simulink model "DCM_speed_control"  (Simulink 7.6)
settings: Solver=ode23tb  StartTime=0.0  StopTime=30  FixedStep=0.0005  MaxStep=1e-4  RelTol=1e-3
values from neighbouring files (symbols this model uses):
  Bm = 0.634    [para_dc.m]
  J = 2.83    [para_dc.m]
  kphi = 4.212    [para_dc.m]
  La = .0065    (= 0.0065)    [para_dc.m]
  Ra = .066    (= 0.066)    [para_dc.m]
  TL = 0    [para_dc.m]
libraries: powerlib_extras x1
settings Model: Creator=DELL  LastModifiedBy=Rhoever  ExtModeTrigMode=oneshot  ExtModeArmWhenConnect=off
settings SolverCC: InitialStep=0.00001
settings DataIOCC: LimitDataPoints=off  SignalLoggingName=sigsOut
settings OptimizationCC: BooleanDataType=off  InitFltsAndDblsToZero=on
settings DebuggingCC: SaveWithParameterizedLinksMsg=none  SignalResolutionControl=TryResolveAllWithWarning  SolverPrmCheckMsg=none  MultiTaskDSMMsg=warning  MultiTaskCondExecSysMsg=none  StrictBusMsg=None
settings HardwareCC: TargetUnknown=on
settings RTWCC: IncludeERTFirstTime=on
settings GRTTargetCC: TargetFcnLib=ansi_tfl_tmw.mat

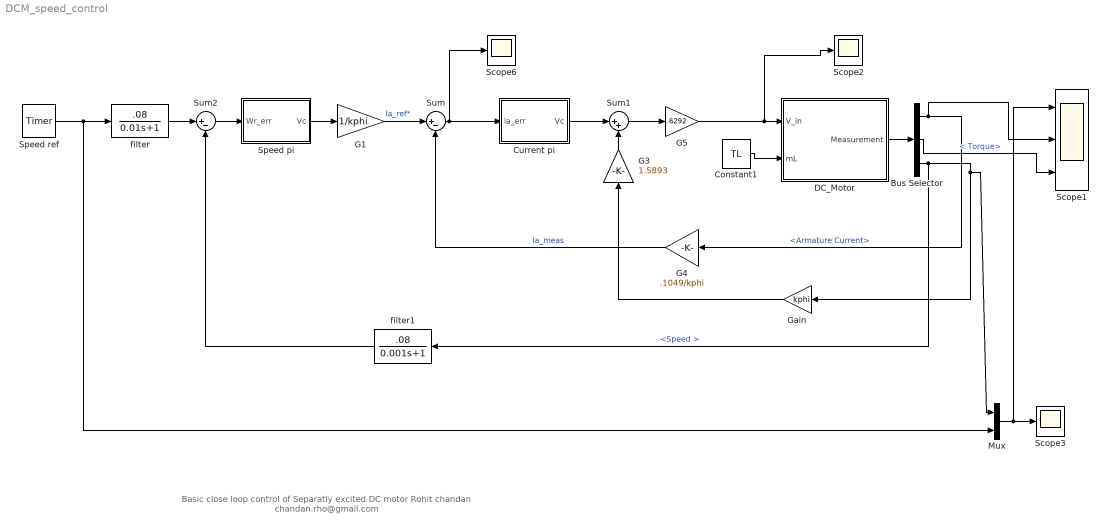
== system DCM_speed_control ==
  note: Basic close loop control of Separatly excited DC motor
      | Rohit chandan
      | chandan.rho@gmail.com
  Bus Selector : BusSelector  OutputSignals=Armature Current, Torque,Speed
  Constant1 : Constant  Value=TL
  Current pi : Subsystem
  DC_Motor : Subsystem
  G1 : Gain  Gain=1/kphi
  G3 : Gain  Gain=1.5893
  G4 : Gain  Gain=.1049/kphi
  G5 : Gain  Gain=.6292
  Gain : Gain  Gain=kphi
  Mux : Mux  Inputs=2
  Scope1 : Scope  NumInputPorts=3
      settings: YMin=2.59672~-5~-5  YMax=2.87006~5~5
  Scope2 : Scope
      settings: YMin=-2.5e+091  YMax=4e+092  SaveName=ScopeData2
  Scope3 : Scope
      settings: TimeRange=4  YMin=-60  YMax=80  SaveName=ScopeData6
  Scope6 : Scope
      settings: YMin=-150  YMax=600  SaveName=ScopeData8
  Speed pi : Subsystem
  Speed ref : powerlib_extras/Control  Blocks/Timer  DialogController=POWERSYS.PowerSysDialog  SystemSampleTime=-1  t=[ 0 7 12 18 25]  e=[80 100 60 -60 80 ]
  Sum : Sum  Inputs=|+-  SaturateOnIntegerOverflow=on  InputSameDT=on  OutDataTypeStr=Inherit: Same as first input
  Sum1 : Sum  Inputs=|++  SaturateOnIntegerOverflow=on  InputSameDT=on  OutDataTypeStr=Inherit: Same as first input
  Sum2 : Sum  Inputs=|+-  SaturateOnIntegerOverflow=on  InputSameDT=on  OutDataTypeStr=Inherit: Same as first input
  filter : TransferFcn  Numerator=[.08]  Denominator=[0.01 1]
  filter1 : TransferFcn  Numerator=[.08]  Denominator=[0.001 1]
  wires:
  Sum/1 -> Scope6/1, Current pi/1(ia_err)
  Mux/1 -> Scope3/1, Scope1/1
  Current pi/1(Vc) -> Sum1/1
  Speed pi/1(Vc) -> G1/1
  Sum2/1 -> Speed pi/1(Wr_err)
  Constant1/1 -> DC_Motor/2(mL)
  Speed ref/1 -> filter/1, Mux/2
  filter/1 -> Sum2/1
  filter1/1 -> Sum2/2
  G3/1 -> Sum1/2
  G1/1 -> Sum/1  "Ia_ref*"
  Sum1/1 -> G5/1
  G5/1 -> DC_Motor/1(V_in), Scope2/1
  G4/1 -> Sum/2  "Ia_meas"
  DC_Motor/1(Measurement) -> Bus Selector/1
  Bus Selector/1 -> G4/1, Scope1/2  "<Armature Current>"
  Bus Selector/3 -> filter1/1, Gain/1, Mux/1  "<Speed >"
  Gain/1 -> G3/1
  Bus Selector/2 -> Scope1/3  "< Torque>"

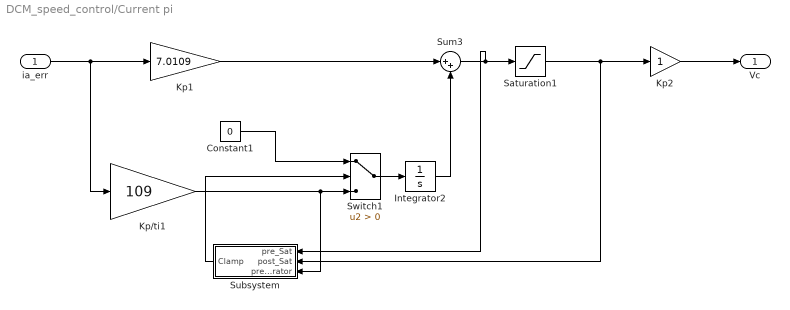
== system DCM_speed_control/Current pi ==
  ia_err : Inport
  Constant1 : Constant  DisableCoverage=on  Value=0  OutDataTypeStr=Inherit: Inherit via back propagation  PreserveConstantTs=on
  Integrator2 : Integrator
  Kp/ti1 : Gain  Gain=109
  Kp1 : Gain  Gain=7.0109
  Kp2 : Gain
  Saturation1 : Saturate  UpperLimit=15  LowerLimit=-15
  Subsystem : Subsystem
  Sum3 : Sum  Inputs=|++
  Switch1 : Switch  DisableCoverage=on  Criteria=u2 > Threshold  InputSameDT=on
  Vc : Outport
  wires:
  Kp1/1 -> Sum3/1
  Sum3/1 -> Saturation1/1, Subsystem/1(pre_Sat)
  Saturation1/1 -> Kp2/1, Subsystem/2(post_Sat)
  ia_err/1 -> Kp1/1, Kp/ti1/1
  Integrator2/1 -> Sum3/2
  Kp/ti1/1 -> Switch1/3, Subsystem/3(pre_Integrator)
  Subsystem/1(Clamp) -> Switch1/2
  Switch1/1 -> Integrator2/1
  Constant1/1 -> Switch1/1
  Kp2/1 -> Vc/1

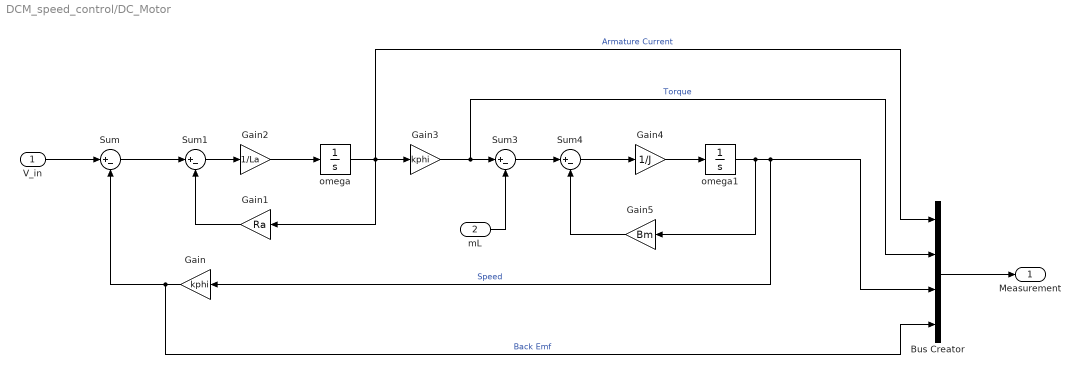
== system DCM_speed_control/DC_Motor ==
  V_in : Inport
  mL : Inport  Port=2
  Bus Creator : BusCreator
  Gain : Gain  Gain=kphi
  Gain1 : Gain  Gain=Ra
  Gain2 : Gain  Gain=1/La
  Gain3 : Gain  Gain=kphi
  Gain4 : Gain  Gain=1/J
  Gain5 : Gain  Gain=Bm
  Sum{,1,3..4} (4 alike) : Sum  Inputs=|+-  SaturateOnIntegerOverflow=on  InputSameDT=on  OutDataTypeStr=Inherit: Same as first input
  omega : Integrator
  omega1 : Integrator
  Measurement : Outport
  wires:
  Sum/1 -> Sum1/1
  V_in/1 -> Sum/1
  Gain/1 -> Sum/2, Bus Creator/4  "Back Emf"
  Gain1/1 -> Sum1/2
  Sum1/1 -> Gain2/1
  Gain2/1 -> omega/1
  omega/1 -> Gain3/1, Gain1/1, Bus Creator/1  "Armature Current"
  Gain3/1 -> Sum3/1, Bus Creator/2  "Torque"
  mL/1 -> Sum3/2
  Sum3/1 -> Sum4/1
  Sum4/1 -> Gain4/1
  Gain4/1 -> omega1/1
  omega1/1 -> Gain5/1, Gain/1, Bus Creator/3  "Speed"
  Gain5/1 -> Sum4/2
  Bus Creator/1 -> Measurement/1

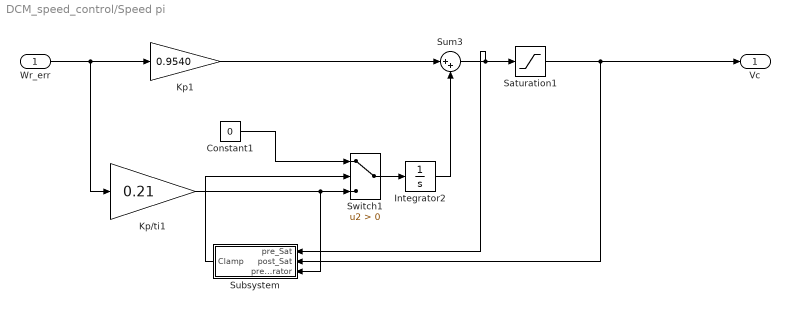
== system DCM_speed_control/Speed pi ==
  Wr_err : Inport
  Constant1 : Constant  DisableCoverage=on  Value=0  OutDataTypeStr=Inherit: Inherit via back propagation  PreserveConstantTs=on
  Integrator2 : Integrator
  Kp/ti1 : Gain  Gain=0.21
  Kp1 : Gain  Gain=0.9540
  Saturation1 : Saturate  UpperLimit=15  LowerLimit=-15
  Subsystem : Subsystem
  Sum3 : Sum  Inputs=|++
  Switch1 : Switch  DisableCoverage=on  Criteria=u2 > Threshold  InputSameDT=on
  Vc : Outport
  wires:
  Constant1/1 -> Switch1/1
  Switch1/1 -> Integrator2/1
  Subsystem/1(Clamp) -> Switch1/2
  Kp/ti1/1 -> Switch1/3, Subsystem/3(pre_Integrator)
  Integrator2/1 -> Sum3/2
  Wr_err/1 -> Kp/ti1/1, Kp1/1
  Saturation1/1 -> Vc/1, Subsystem/2(post_Sat)
  Sum3/1 -> Saturation1/1, Subsystem/1(pre_Sat)
  Kp1/1 -> Sum3/1

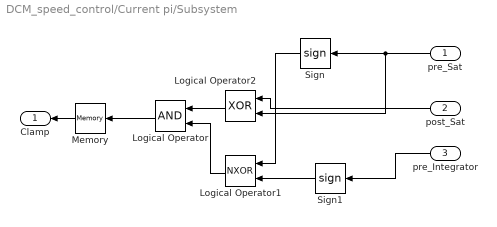
== system DCM_speed_control/Current pi/Subsystem ==
  pre_Sat : Inport
  post_Sat : Inport  Port=2
  pre_Integrator : Inport  Port=3
  Logical Operator : Logic  AllPortsSameDT=off  OutDataTypeStr=boolean
  Logical Operator1 : Logic  Operator=NXOR  AllPortsSameDT=off  OutDataTypeStr=boolean
  Logical Operator2 : Logic  Operator=XOR  AllPortsSameDT=off  OutDataTypeStr=boolean
  Memory : Memory
  Sign : Signum
  Sign1 : Signum
  Clamp : Outport
  wires:
  Logical Operator/1 -> Memory/1
  Logical Operator2/1 -> Logical Operator/1
  Logical Operator1/1 -> Logical Operator/2
  Sign/1 -> Logical Operator1/1
  Sign1/1 -> Logical Operator1/2
  Memory/1 -> Clamp/1
  pre_Sat/1 -> Sign/1, Logical Operator2/2
  post_Sat/1 -> Logical Operator2/1
  pre_Integrator/1 -> Sign1/1

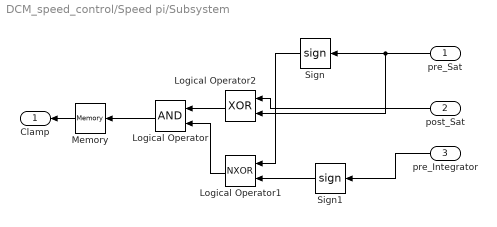
== system DCM_speed_control/Speed pi/Subsystem ==
  pre_Sat : Inport
  post_Sat : Inport  Port=2
  pre_Integrator : Inport  Port=3
  Logical Operator : Logic  AllPortsSameDT=off  OutDataTypeStr=boolean
  Logical Operator1 : Logic  Operator=NXOR  AllPortsSameDT=off  OutDataTypeStr=boolean
  Logical Operator2 : Logic  Operator=XOR  AllPortsSameDT=off  OutDataTypeStr=boolean
  Memory : Memory
  Sign : Signum
  Sign1 : Signum
  Clamp : Outport
  wires:
  Logical Operator/1 -> Memory/1
  Logical Operator2/1 -> Logical Operator/1
  Logical Operator1/1 -> Logical Operator/2
  Sign/1 -> Logical Operator1/1
  Sign1/1 -> Logical Operator1/2
  Memory/1 -> Clamp/1
  pre_Sat/1 -> Sign/1, Logical Operator2/2
  post_Sat/1 -> Logical Operator2/1
  pre_Integrator/1 -> Sign1/1
